simulink model "pendulum"  (R2013b)
settings: Solver=ode45  StartTime=0.0  StopTime=10  RelTol=1e-3
undefined symbols (not defined in the file or in its folder): dT
settings Model: Creator=igeorgie  LastModifiedBy=igeorgie

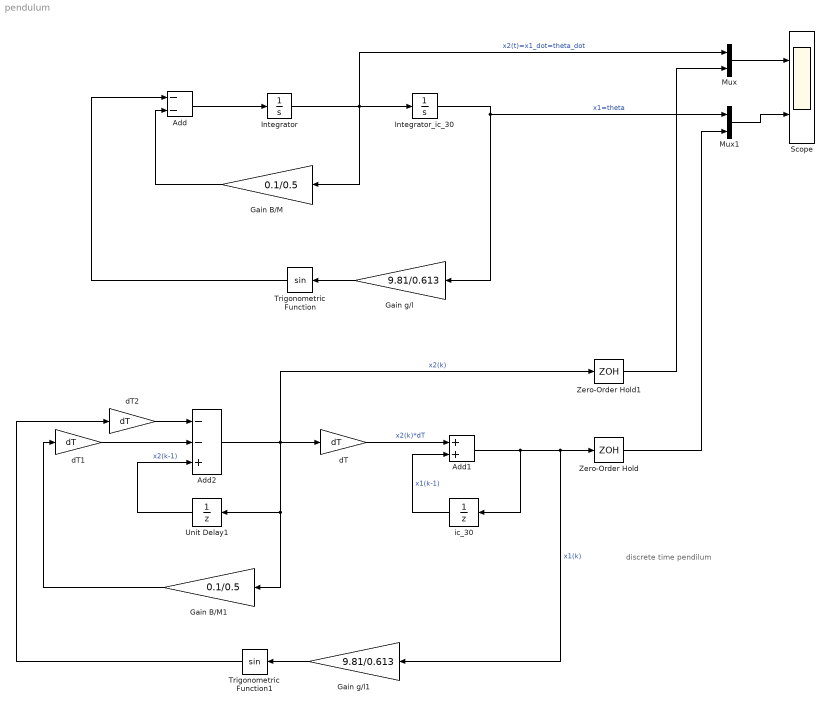
== system pendulum ==
  note: discrete time pendilum
  Add : Sum  Inputs=--
  Add1 : Sum
  Add2 : Sum  Inputs=--+
  Gain B/M : Gain  Gain=0.1/0.5
  Gain B/M1 : Gain  Gain=0.1/0.5
  Gain g/l : Gain  Gain=9.81/0.613
  Gain g/l1 : Gain  Gain=9.81/0.613
  Integrator : Integrator
  Integrator_ic_30 : Integrator  InitialCondition=0.5
  Mux : Mux  Inputs=2
  Mux1 : Mux  Inputs=2
  Scope : Scope  NumInputPorts=2
      settings: YMin=-5~-5  YMax=5~5
  Trigonometric Function : Trigonometry
  Trigonometric Function1 : Trigonometry
  Unit Delay1 : UnitDelay  SampleTime=-1
  Zero-Order Hold : ZeroOrderHold  SampleTime=dT
  Zero-Order Hold1 : ZeroOrderHold  SampleTime=dT
  dT : Gain  Gain=dT
  dT1 : Gain  Gain=dT
  dT2 : Gain  Gain=dT
  ic_30 : UnitDelay  InitialCondition=0.5  SampleTime=-1
  wires:
  Add/1 -> Integrator/1
  Gain B/M/1 -> Add/2
  Integrator/1 -> Mux/1, Gain B/M/1, Integrator_ic_30/1  "x2(t)=x1_dot=theta_dot"
  Trigonometric Function/1 -> Add/1
  Gain g/l/1 -> Trigonometric Function/1
  Integrator_ic_30/1 -> Mux1/1, Gain g/l/1  "x1=theta"
  Add1/1 -> Zero-Order Hold/1, Gain g/l1/1, ic_30/1  "x1(k)"
  Add2/1 -> Zero-Order Hold1/1, Gain B/M1/1, Unit Delay1/1, dT/1  "x2(k)"
  ic_30/1 -> Add1/2  "x1(k-1)"
  dT/1 -> Add1/1  "x2(k)*dT"
  Unit Delay1/1 -> Add2/3  "x2(k-1)"
  dT1/1 -> Add2/2
  Gain B/M1/1 -> dT1/1
  Gain g/l1/1 -> Trigonometric Function1/1
  Trigonometric Function1/1 -> dT2/1
  Zero-Order Hold/1 -> Mux1/2
  dT2/1 -> Add2/1
  Mux/1 -> Scope/1
  Zero-Order Hold1/1 -> Mux/2
  Mux1/1 -> Scope/2
